simulink model "FFM_Punch"  (R2017a)
settings: Solver=ode3  StartTime=0.0  StopTime=timesteps  FixedStep=data.SIM.Ts  RelTol=1e-3  EnableMultiTasking=on
values from neighbouring files (symbols this model uses):
  data =     [dakota_config.mat]
  downshift_map = data.TCU.upshift.veh_spd_default    [Simulation_results.m]
  upshift_map = data.TCU.upshift.veh_spd_default    [Simulation_results.m]
undefined symbols (not defined in the file or in its folder): air_density, Cd, DiscIntNeverNeededParam, fr_crankshaft, fr_speed_values, g, i_FD, ICE, Low_Ratio, M_Eng_Max, M_Eng_Max_Max, M_Eng_Max_Rpm, mt2m_f, mu_Roll_C0, mu_Roll_C1, mu_Roll_C2, Mv, n_Idle_Eng, Overdrive_Ratio, Re, S_eff_drag, Ts
(part 15 of 15)

== system FFM_Punch/Driver Interface/Driver Model/Driver Pedals Determination/Throttle_Pedal_Determination/RateLimiter ==
  UL : Inport  Tag=Controls_Lib_V1.0  OutDataTypeStr=single  Interpolate=off
  Inp : Inport  Tag=Controls_Lib_V1.0  Port=2  OutDataTypeStr=single  Interpolate=off
  LL : Inport  Tag=Controls_Lib_V1.0  Port=3  OutDataTypeStr=single  Interpolate=off
  AddSub : Sum  Tag=Controls_Lib_V1.0  Inputs=+-  CollapseDim=CollapseDim  AccumDataTypeStr=single  OutMin=OutMin  OutMax=OutMax  OutDataTypeStr=single  RndMeth=Nearest  SampleTime=SampleTime  InputSameDT=on  mask(AddSub){IconShape=rectangular, Inputs=+-, CollapseMode=All dimensions, CollapseDim=1, SampleTime=-1, InputSameDT=on, AccumDataTypeStr=single, OutMin=[], OutMax=[], OutDataTypeStr=single, LockScale=off, RndMeth=Nearest, SaturateOnIntegerOverflow=off}
      mask prompts: IconShape "Icon shape:"; Inputs "List of signs:"; CollapseMode "Sum over:"; CollapseDim "Dimension:"; SampleTime "Sample time (-1 for inherited):"; InputSameDT "Require all inputs to have the same data type"; AccumDataTypeStr "Accumulator data type:"; OutMin "Output minimum:"; OutMax "Output maximum:"; OutDataTypeStr "Output data type:"; LockScale "Lock data type settings against changes by the fixed-point tools"; RndMeth "Integer rounding mode:"; SaturateOnIntegerOverflow "Saturate on integer overflow"
      mask help:
      | Add or subtract inputs.  Specify one of the following:
      | a) string containing + or - for each input port, | for spacer between ports (e.g. ++|-|++)
      | b) scalar, >= 1, specifies the number of input ports to be summed.
      | When there is only one input port, add or subtract elements over all dimensions or one specified dimension
      mask Help: web([fileparts(which('Lib_built')) filesep 'hlp' filesep 'lib_AddSub' '.html'], '-helpbrowser')
      mask TypeOptions IconShape: IconShape
      mask TypeOptions Inputs: Inputs
      mask TypeOptions CollapseMode: CollapseMode
      mask TypeOptions CollapseDim: CollapseDim
      mask TypeOptions SampleTime: SampleTime
      mask TypeOptions InputSameDT: InputSameDT
      mask TypeOptions AccumDataTypeStr: AccumDataTypeStr
      mask TypeOptions OutMin: OutMin
      mask TypeOptions OutMax: OutMax
      mask TypeOptions OutDataTypeStr: OutDataTypeStr
      mask TypeOptions LockScale: LockScale
      mask TypeOptions RndMeth: RndMeth
      mask TypeOptions SaturateOnIntegerOverflow: SaturateOnIntegerOverflow
  AddSub1 : Sum  Tag=Controls_Lib_V1.0  CollapseDim=CollapseDim  AccumDataTypeStr=single  OutMin=OutMin  OutMax=OutMax  OutDataTypeStr=single  RndMeth=Nearest  SampleTime=SampleTime  InputSameDT=on  mask(AddSub){IconShape=rectangular, Inputs=++, CollapseMode=All dimensions, CollapseDim=1, SampleTime=-1, InputSameDT=on, AccumDataTypeStr=single, OutMin=[], OutMax=[], OutDataTypeStr=single, LockScale=off, RndMeth=Nearest, SaturateOnIntegerOverflow=off}
      mask prompts: IconShape "Icon shape:"; Inputs "List of signs:"; CollapseMode "Sum over:"; CollapseDim "Dimension:"; SampleTime "Sample time (-1 for inherited):"; InputSameDT "Require all inputs to have the same data type"; AccumDataTypeStr "Accumulator data type:"; OutMin "Output minimum:"; OutMax "Output maximum:"; OutDataTypeStr "Output data type:"; LockScale "Lock data type settings against changes by the fixed-point tools"; RndMeth "Integer rounding mode:"; SaturateOnIntegerOverflow "Saturate on integer overflow"
      mask help:
      | Add or subtract inputs.  Specify one of the following:
      | a) string containing + or - for each input port, | for spacer between ports (e.g. ++|-|++)
      | b) scalar, >= 1, specifies the number of input ports to be summed.
      | When there is only one input port, add or subtract elements over all dimensions or one specified dimension
      mask Help: web([fileparts(which('Lib_built')) filesep 'hlp' filesep 'lib_AddSub' '.html'], '-helpbrowser')
      mask TypeOptions IconShape: IconShape
      mask TypeOptions Inputs: Inputs
      mask TypeOptions CollapseMode: CollapseMode
      mask TypeOptions CollapseDim: CollapseDim
      mask TypeOptions SampleTime: SampleTime
      mask TypeOptions InputSameDT: InputSameDT
      mask TypeOptions AccumDataTypeStr: AccumDataTypeStr
      mask TypeOptions OutMin: OutMin
      mask TypeOptions OutMax: OutMax
      mask TypeOptions OutDataTypeStr: OutDataTypeStr
      mask TypeOptions LockScale: LockScale
      mask TypeOptions RndMeth: RndMeth
      mask TypeOptions SaturateOnIntegerOverflow: SaturateOnIntegerOverflow
  AddSub2 : Sum  Tag=Controls_Lib_V1.0  CollapseDim=CollapseDim  AccumDataTypeStr=single  OutMin=OutMin  OutMax=OutMax  OutDataTypeStr=single  RndMeth=Nearest  SampleTime=SampleTime  InputSameDT=on  mask(AddSub){IconShape=rectangular, Inputs=++, CollapseMode=All dimensions, CollapseDim=1, SampleTime=-1, InputSameDT=on, AccumDataTypeStr=single, OutMin=[], OutMax=[], OutDataTypeStr=single, LockScale=off, RndMeth=Nearest, SaturateOnIntegerOverflow=off}
      mask prompts: IconShape "Icon shape:"; Inputs "List of signs:"; CollapseMode "Sum over:"; CollapseDim "Dimension:"; SampleTime "Sample time (-1 for inherited):"; InputSameDT "Require all inputs to have the same data type"; AccumDataTypeStr "Accumulator data type:"; OutMin "Output minimum:"; OutMax "Output maximum:"; OutDataTypeStr "Output data type:"; LockScale "Lock data type settings against changes by the fixed-point tools"; RndMeth "Integer rounding mode:"; SaturateOnIntegerOverflow "Saturate on integer overflow"
      mask help:
      | Add or subtract inputs.  Specify one of the following:
      | a) string containing + or - for each input port, | for spacer between ports (e.g. ++|-|++)
      | b) scalar, >= 1, specifies the number of input ports to be summed.
      | When there is only one input port, add or subtract elements over all dimensions or one specified dimension
      mask Help: web([fileparts(which('Lib_built')) filesep 'hlp' filesep 'lib_AddSub' '.html'], '-helpbrowser')
      mask TypeOptions IconShape: IconShape
      mask TypeOptions Inputs: Inputs
      mask TypeOptions CollapseMode: CollapseMode
      mask TypeOptions CollapseDim: CollapseDim
      mask TypeOptions SampleTime: SampleTime
      mask TypeOptions InputSameDT: InputSameDT
      mask TypeOptions AccumDataTypeStr: AccumDataTypeStr
      mask TypeOptions OutMin: OutMin
      mask TypeOptions OutMax: OutMax
      mask TypeOptions OutDataTypeStr: OutDataTypeStr
      mask TypeOptions LockScale: LockScale
      mask TypeOptions RndMeth: RndMeth
      mask TypeOptions SaturateOnIntegerOverflow: SaturateOnIntegerOverflow
  AddSub3 : Sum  Tag=Controls_Lib_V1.0  Inputs=-+  CollapseDim=CollapseDim  AccumDataTypeStr=single  OutMin=OutMin  OutMax=OutMax  OutDataTypeStr=single  RndMeth=Nearest  SampleTime=SampleTime  InputSameDT=on  mask(AddSub){IconShape=rectangular, Inputs=-+, CollapseMode=All dimensions, CollapseDim=1, SampleTime=-1, InputSameDT=on, AccumDataTypeStr=single, OutMin=[], OutMax=[], OutDataTypeStr=single, LockScale=off, RndMeth=Nearest, SaturateOnIntegerOverflow=off}
      mask prompts: IconShape "Icon shape:"; Inputs "List of signs:"; CollapseMode "Sum over:"; CollapseDim "Dimension:"; SampleTime "Sample time (-1 for inherited):"; InputSameDT "Require all inputs to have the same data type"; AccumDataTypeStr "Accumulator data type:"; OutMin "Output minimum:"; OutMax "Output maximum:"; OutDataTypeStr "Output data type:"; LockScale "Lock data type settings against changes by the fixed-point tools"; RndMeth "Integer rounding mode:"; SaturateOnIntegerOverflow "Saturate on integer overflow"
      mask help:
      | Add or subtract inputs.  Specify one of the following:
      | a) string containing + or - for each input port, | for spacer between ports (e.g. ++|-|++)
      | b) scalar, >= 1, specifies the number of input ports to be summed.
      | When there is only one input port, add or subtract elements over all dimensions or one specified dimension
      mask Help: web([fileparts(which('Lib_built')) filesep 'hlp' filesep 'lib_AddSub' '.html'], '-helpbrowser')
      mask TypeOptions IconShape: IconShape
      mask TypeOptions Inputs: Inputs
      mask TypeOptions CollapseMode: CollapseMode
      mask TypeOptions CollapseDim: CollapseDim
      mask TypeOptions SampleTime: SampleTime
      mask TypeOptions InputSameDT: InputSameDT
      mask TypeOptions AccumDataTypeStr: AccumDataTypeStr
      mask TypeOptions OutMin: OutMin
      mask TypeOptions OutMax: OutMax
      mask TypeOptions OutDataTypeStr: OutDataTypeStr
      mask TypeOptions LockScale: LockScale
      mask TypeOptions RndMeth: RndMeth
      mask TypeOptions SaturateOnIntegerOverflow: SaturateOnIntegerOverflow
  Constant : Constant  Tag=Controls_Lib_V1.0  Value=Value  VectorParams1D=off  OutMin=OutMin  OutMax=OutMax  OutDataTypeStr=Inherit: Inherit via back propagation  SampleTime=SampleTime  FramePeriod=FramePeriod  mask(Constant){Value=0.5, VectorParams1D=off, SampleTime=-1, FramePeriod=inf, OutMin=[], OutMax=[], OutDataTypeStr=Inherit: Inherit via back propagation, LockScale=off}
      mask prompts: Value "Constant value:"; VectorParams1D "Interpret vector parameters as 1-D"; SampleTime "Sample time:"; FramePeriod "Frame period:"; OutMin "Output minimum:"; OutMax "Output maximum:"; OutDataTypeStr "Output data type:"; LockScale "Lock output data type setting against changes by the fixed-point tools"
      mask help: Output the constant specified by the 'Constant value' parameter.
      mask TypeOptions Value: Value
      mask TypeOptions VectorParams1D: VectorParams1D
      mask TypeOptions SampleTime: SampleTime
      mask TypeOptions FramePeriod: FramePeriod
      mask TypeOptions OutMin: OutMin
      mask TypeOptions OutMax: OutMax
      mask TypeOptions OutDataTypeStr: OutDataTypeStr
      mask TypeOptions LockScale: LockScale
      mask Display: disp(get_param(gcb,'Value'))
  Constant1 : Constant  Tag=Controls_Lib  Description=constant  Value=Value  OutMin=OutMin  OutMax=OutMax  OutDataTypeStr=single  SampleTime=SampleTime  FramePeriod=FramePeriod  mask(Constant){Value=1, VectorParams1D=on, SampleTime=-1, FramePeriod=inf, OutMin=[], OutMax=[], OutDataTypeStr=single, LockScale=off}
      mask prompts: Value "Constant value:"; VectorParams1D "Interpret vector parameters as 1-D"; SampleTime "Sample time:"; FramePeriod "Frame period:"; OutMin "Output minimum:"; OutMax "Output maximum:"; OutDataTypeStr "Output data type:"; LockScale "Lock output data type setting against changes by the fixed-point tools"
      mask help: Output the constant specified by the 'Constant value' parameter.
      mask TypeOptions Value: Value
      mask TypeOptions VectorParams1D: VectorParams1D
      mask TypeOptions SampleTime: SampleTime
      mask TypeOptions FramePeriod: FramePeriod
      mask TypeOptions OutMin: OutMin
      mask TypeOptions OutMax: OutMax
      mask TypeOptions OutDataTypeStr: OutDataTypeStr
      mask TypeOptions LockScale: LockScale
      mask Display: disp(get_param(gcb,'Value'))
  Delay : Delay  Tag=Controls_Lib_V1.0  DelayLength=DelayLength  DelayLengthUpperLimit=DelayLengthUpperLimit  InitialConditionSource=Input port  InitialCondition=InitialCondition  SampleTime=SampleTime  mask(Delay){DelayLengthSource=Dialog, DelayLength=1, DelayLengthUpperLimit=100, InitialConditionSource=Input port, InitialCondition=0.0, ExternalReset=None, PreventDirectFeedthrough=off, DiagnosticForOutOfRangeDelayLength=None, RemoveProtectionDelayLength=off, InputProcessing=Elements as channels (sample based), UseCircularBuffer=off, SampleTime=-1, StateName=, StateMustResolveToSignalObject=off, CodeGenStateStorageClass=Auto, CodeGenStateStorageTypeQualifier=}
      mask prompts: DelayLengthSource "Delay length source:"; DelayLength "Delay length:"; DelayLengthUpperLimit "Delay upper limit:"; InitialConditionSource "Initial condition source:"; InitialCondition "Initial condition:"; ExternalReset "External reset:"; PreventDirectFeedthrough "Prevent direct feedthrough by increasing delay length to lower limit"; DiagnosticForOutOfRangeDelayLength "Diagnostic for out-of-range delay length:"; RemoveProtectionDelayLength "Remove protection against out-of-range delay length in generated code"; InputProcessing "Input processing:"; UseCircularBuffer "Use circular buffer for state"; SampleTime "Sample time (-1 for inherited):"; StateName "State name:"; StateMustResolveToSignalObject "State name must resolve to Simulink signal object"; CodeGenStateStorageClass "Code generation storage class:"; CodeGenStateStorageTypeQualifier "Code generation storage type qualifier:"
      mask help: Delay input by a fixed or variable number of samples. The initial output of the delay block is specified by the external input x0.
      settings: InputPortMap=u0,p4
      mask TypeOptions DelayLengthSource: DelayLengthSource
      mask TypeOptions DelayLength: DelayLength
      mask TypeOptions DelayLengthUpperLimit: DelayLengthUpperLimit
      mask TypeOptions InitialConditionSource: InitialConditionSource
      mask TypeOptions InitialCondition: InitialCondition
      mask TypeOptions ExternalReset: ExternalReset
      mask TypeOptions PreventDirectFeedthrough: PreventDirectFeedthrough
      mask TypeOptions DiagnosticForOutOfRangeDelayLength: DiagnosticForOutOfRangeDelayLength
      mask TypeOptions RemoveProtectionDelayLength: RemoveProtectionDelayLength
      mask TypeOptions InputProcessing: InputProcessing
      mask TypeOptions UseCircularBuffer: UseCircularBuffer
      mask TypeOptions SampleTime: SampleTime
      mask TypeOptions StateName: StateName
      mask TypeOptions StateMustResolveToSignalObject: StateMustResolveToSignalObject
      mask TypeOptions CodeGenStateStorageClass: CodeGenStateStorageClass
      mask TypeOptions CodeGenStateStorageTypeQualifier: CodeGenStateStorageTypeQualifier
  MulDiv : Product  Tag=Controls_Lib_V1.0  Inputs=*/  CollapseDim=CollapseDim  OutMin=OutMin  OutMax=OutMax  OutDataTypeStr=single  SampleTime=SampleTime  InputSameDT=on  mask(MulDiv){Inputs=*/, Multiplication=Element-wise(.*), CollapseMode=All dimensions, CollapseDim=1, SampleTime=-1, InputSameDT=on, OutMin=[], OutMax=[], OutDataTypeStr=single, LockScale=off, RndMeth=Floor, SaturateOnIntegerOverflow=off}
      mask prompts: Inputs "Number of inputs:"; CollapseMode "Multiply over:"; CollapseDim "Dimension:"; SampleTime "Sample time (-1 for inherited):"; InputSameDT "Require all inputs to have the same data type"; OutMin "Output minimum:"; OutMax "Output maximum:"; OutDataTypeStr "Output data type:"; LockScale "Lock output data type setting against changes by the fixed-point tools"; RndMeth "Integer rounding mode:"; SaturateOnIntegerOverflow "Saturate on integer overflow"
      mask help:
      | Multiply or divide inputs element-wise. Specify one of the following:
      |  a) * or / for each input port. For example, **/* performs the operation 'u1*u2/u3*u4'.
      |  b) scalar specifies the number of input ports to be multiplied.
      | If there is only one input port and the Multiplication parameter is set to Element-wise(.*), a single * or / collapses the input signal using the specified operation.
      mask Help: web([fileparts(which('Lib_built')) filesep 'hlp' filesep 'lib_MulDiv' '.html'], '-helpbrowser')
      mask TypeOptions Inputs: Inputs
      mask TypeOptions Multiplication: Multiplication
      mask TypeOptions CollapseMode: CollapseMode
      mask TypeOptions CollapseDim: CollapseDim
      mask TypeOptions SampleTime: SampleTime
      mask TypeOptions InputSameDT: InputSameDT
      mask TypeOptions OutMin: OutMin
      mask TypeOptions OutMax: OutMax
      mask TypeOptions OutDataTypeStr: OutDataTypeStr
      mask TypeOptions LockScale: LockScale
      mask TypeOptions RndMeth: RndMeth
      mask TypeOptions SaturateOnIntegerOverflow: SaturateOnIntegerOverflow
  MulDiv1 : Product  Tag=Controls_Lib_V1.0  Inputs=**  CollapseDim=CollapseDim  OutMin=OutMin  OutMax=OutMax  OutDataTypeStr=single  SampleTime=SampleTime  InputSameDT=on  mask(MulDiv){Inputs=**, Multiplication=Element-wise(.*), CollapseMode=All dimensions, CollapseDim=1, SampleTime=-1, InputSameDT=on, OutMin=[], OutMax=[], OutDataTypeStr=single, LockScale=off, RndMeth=Floor, SaturateOnIntegerOverflow=off}
      mask prompts: Inputs "Number of inputs:"; CollapseMode "Multiply over:"; CollapseDim "Dimension:"; SampleTime "Sample time (-1 for inherited):"; InputSameDT "Require all inputs to have the same data type"; OutMin "Output minimum:"; OutMax "Output maximum:"; OutDataTypeStr "Output data type:"; LockScale "Lock output data type setting against changes by the fixed-point tools"; RndMeth "Integer rounding mode:"; SaturateOnIntegerOverflow "Saturate on integer overflow"
      mask help:
      | Multiply or divide inputs element-wise. Specify one of the following:
      |  a) * or / for each input port. For example, **/* performs the operation 'u1*u2/u3*u4'.
      |  b) scalar specifies the number of input ports to be multiplied.
      | If there is only one input port and the Multiplication parameter is set to Element-wise(.*), a single * or / collapses the input signal using the specified operation.
      mask Help: web([fileparts(which('Lib_built')) filesep 'hlp' filesep 'lib_MulDiv' '.html'], '-helpbrowser')
      mask TypeOptions Inputs: Inputs
      mask TypeOptions Multiplication: Multiplication
      mask TypeOptions CollapseMode: CollapseMode
      mask TypeOptions CollapseDim: CollapseDim
      mask TypeOptions SampleTime: SampleTime
      mask TypeOptions InputSameDT: InputSameDT
      mask TypeOptions OutMin: OutMin
      mask TypeOptions OutMax: OutMax
      mask TypeOptions OutDataTypeStr: OutDataTypeStr
      mask TypeOptions LockScale: LockScale
      mask TypeOptions RndMeth: RndMeth
      mask TypeOptions SaturateOnIntegerOverflow: SaturateOnIntegerOverflow
  MulDiv2 : Product  Tag=Controls_Lib_V1.0  Inputs=***  CollapseDim=CollapseDim  OutMin=OutMin  OutMax=OutMax  OutDataTypeStr=single  SampleTime=SampleTime  InputSameDT=on  mask(MulDiv){Inputs=***, Multiplication=Element-wise(.*), CollapseMode=All dimensions, CollapseDim=1, SampleTime=-1, InputSameDT=on, OutMin=[], OutMax=[], OutDataTypeStr=single, LockScale=off, RndMeth=Floor, SaturateOnIntegerOverflow=off}
      mask prompts: Inputs "Number of inputs:"; CollapseMode "Multiply over:"; CollapseDim "Dimension:"; SampleTime "Sample time (-1 for inherited):"; InputSameDT "Require all inputs to have the same data type"; OutMin "Output minimum:"; OutMax "Output maximum:"; OutDataTypeStr "Output data type:"; LockScale "Lock output data type setting against changes by the fixed-point tools"; RndMeth "Integer rounding mode:"; SaturateOnIntegerOverflow "Saturate on integer overflow"
      mask help:
      | Multiply or divide inputs element-wise. Specify one of the following:
      |  a) * or / for each input port. For example, **/* performs the operation 'u1*u2/u3*u4'.
      |  b) scalar specifies the number of input ports to be multiplied.
      | If there is only one input port and the Multiplication parameter is set to Element-wise(.*), a single * or / collapses the input signal using the specified operation.
      mask Help: web([fileparts(which('Lib_built')) filesep 'hlp' filesep 'lib_MulDiv' '.html'], '-helpbrowser')
      mask TypeOptions Inputs: Inputs
      mask TypeOptions Multiplication: Multiplication
      mask TypeOptions CollapseMode: CollapseMode
      mask TypeOptions CollapseDim: CollapseDim
      mask TypeOptions SampleTime: SampleTime
      mask TypeOptions InputSameDT: InputSameDT
      mask TypeOptions OutMin: OutMin
      mask TypeOptions OutMax: OutMax
      mask TypeOptions OutDataTypeStr: OutDataTypeStr
      mask TypeOptions LockScale: LockScale
      mask TypeOptions RndMeth: RndMeth
      mask TypeOptions SaturateOnIntegerOverflow: SaturateOnIntegerOverflow
  MulDiv3 : Product  Tag=Controls_Lib_V1.0  Inputs=*/  CollapseDim=CollapseDim  OutMin=OutMin  OutMax=OutMax  OutDataTypeStr=single  SampleTime=SampleTime  InputSameDT=on  mask(MulDiv){Inputs=*/, Multiplication=Element-wise(.*), CollapseMode=All dimensions, CollapseDim=1, SampleTime=-1, InputSameDT=on, OutMin=[], OutMax=[], OutDataTypeStr=single, LockScale=off, RndMeth=Floor, SaturateOnIntegerOverflow=off}
      mask prompts: Inputs "Number of inputs:"; CollapseMode "Multiply over:"; CollapseDim "Dimension:"; SampleTime "Sample time (-1 for inherited):"; InputSameDT "Require all inputs to have the same data type"; OutMin "Output minimum:"; OutMax "Output maximum:"; OutDataTypeStr "Output data type:"; LockScale "Lock output data type setting against changes by the fixed-point tools"; RndMeth "Integer rounding mode:"; SaturateOnIntegerOverflow "Saturate on integer overflow"
      mask help:
      | Multiply or divide inputs element-wise. Specify one of the following:
      |  a) * or / for each input port. For example, **/* performs the operation 'u1*u2/u3*u4'.
      |  b) scalar specifies the number of input ports to be multiplied.
      | If there is only one input port and the Multiplication parameter is set to Element-wise(.*), a single * or / collapses the input signal using the specified operation.
      mask Help: web([fileparts(which('Lib_built')) filesep 'hlp' filesep 'lib_MulDiv' '.html'], '-helpbrowser')
      mask TypeOptions Inputs: Inputs
      mask TypeOptions Multiplication: Multiplication
      mask TypeOptions CollapseMode: CollapseMode
      mask TypeOptions CollapseDim: CollapseDim
      mask TypeOptions SampleTime: SampleTime
      mask TypeOptions InputSameDT: InputSameDT
      mask TypeOptions OutMin: OutMin
      mask TypeOptions OutMax: OutMax
      mask TypeOptions OutDataTypeStr: OutDataTypeStr
      mask TypeOptions LockScale: LockScale
      mask TypeOptions RndMeth: RndMeth
      mask TypeOptions SaturateOnIntegerOverflow: SaturateOnIntegerOverflow
  SatChck : Subsystem  mask(SATURATION){}
      mask help:
      | The Saturation with Check block imposes upper and lower limits on an input signal. If the input signal is outside of these limits, saturation flag shall be raised.
      |
      | The upper limit (Max) shall be  greater than the lower limit (Min) for the saturation block to work as intended.
      mask Help: web([fileparts(which('Lib_discontious')) filesep 'hlp' filesep 'lib_SatChck.html'], '-helpbrowser')
      mask Display: plot([0 1 2 3 4 5],[0 0 0 1 1 1],[0 5],[0.5 0.5],[2.5 2.5],[0 1])
  TsInverse : SampleTimeMath  TsampMathOp=1/Ts Only  weightValue=weightValue  OutDataTypeStr=Inherit: Inherit via back propagation  mask(Sample time block){TsampMathOp=1/Ts Only, weightValue=1, TsampMathImp=Online Calculations, OutDataTypeStr=Inherit: Inherit via back propagation, RndMeth=Floor, SaturateOnIntegerOverflow=off}
      mask prompts: TsampMathOp "Operation:"; weightValue "Weight value:"; TsampMathImp "Implement using:"; OutDataTypeStr "Output data type:"; RndMeth "Integer rounding mode:"; SaturateOnIntegerOverflow "Saturate on integer overflow"
      mask help: 1 divided by the Sample time of the input signal
      mask Help: web([fileparts(which('Lib_built')) filesep 'hlp' filesep 'lib_TsInv' '.html'], '-helpbrowser')
      mask TypeOptions TsampMathOp: TsampMathOp
      mask TypeOptions weightValue: weightValue
      mask TypeOptions TsampMathImp: TsampMathImp
      mask TypeOptions OutDataTypeStr: OutDataTypeStr
      mask TypeOptions RndMeth: RndMeth
      mask TypeOptions SaturateOnIntegerOverflow: SaturateOnIntegerOverflow
  Out : Outport  Tag=Controls_Lib_V1.0  OutDataTypeStr=single  InitialOutput=0
  Issat : Outport  Tag=Controls_Lib_V1.0  Port=2  OutDataTypeStr=boolean  InitialOutput=0
  wires:
  MulDiv3/1 -> [Ts]
  TsInverse/1 -> MulDiv3/2
  Constant1/1 -> MulDiv3/1
  [Init] -> Delay/2
  Delay/1 -> [OutPrev]
  AddSub3/1 -> [Init]
  MulDiv2/1 -> AddSub3/1
  [Inp] -> AddSub3/2
  Constant/1 -> MulDiv2/3
  AddSub2/1 -> MulDiv2/2
  [LL] -> AddSub2/2
  [UL] -> AddSub2/1
  AddSub1/1 -> Delay/1, Out/1
  [Ts] -> MulDiv1/1
  [OutPrev] -> AddSub1/2
  MulDiv1/1 -> AddSub1/1
  SatChck/1(ValSat) -> MulDiv1/2
  MulDiv/1 -> SatChck/2(Inp)
  [Ts] -> MulDiv2/1, MulDiv/2
  AddSub/1 -> MulDiv/1
  SatChck/2(IsSat) -> Issat/1
  [LL] -> SatChck/3(Min)
  [UL] -> SatChck/1(Max)
  [OutPrev] -> AddSub/2
  [Inp] -> AddSub/1
  LL/1 -> [LL]
  Inp/1 -> TsInverse/1, [Inp]
  UL/1 -> [UL]

== system FFM_Punch/Driver Interface/Driver Model/Final Pedal Coordination/RateLimiter/SatChck ==
  Max : Inport  Tag=Controls_Lib_V1.0  OutDataTypeStr=single  Interpolate=off
  Inp : Inport  Tag=Controls_Lib_V1.0  Port=2  OutDataTypeStr=single  Interpolate=off
  Min : Inport  Tag=Controls_Lib_V1.0  Port=3  OutDataTypeStr=single  Interpolate=off
  MinMax : MinMax  Tag=Controls_Lib_V1.0  Inputs=Inputs  OutMin=OutMin  OutMax=OutMax  OutDataTypeStr=single  RndMeth=Zero  SampleTime=SampleTime  InputSameDT=on  mask(MinMax){Function=min, Inputs=2, ZeroCross=on, SampleTime=-1, InputSameDT=on, OutMin=[], OutMax=[], OutDataTypeStr=single, LockScale=off, RndMeth=Zero, SaturateOnIntegerOverflow=off}
      mask prompts: Inputs "Number of input ports:"; ZeroCross "Enable zero-crossing detection"; SampleTime "Sample time (-1 for inherited):"; InputSameDT "Require all inputs to have the same data type"; OutMin "Output minimum:"; OutMax "Output maximum:"; OutDataTypeStr "Output data type:"; LockScale "Lock output data type setting against changes by the fixed-point tools"; RndMeth "Integer rounding mode:"; SaturateOnIntegerOverflow "Saturate on integer overflow"
      mask help: Output min or max of input. For a single input, operators are applied across the input vector. For multiple inputs, operators are applied across the inputs.
      mask Help: web([fileparts(which('Lib_built')) filesep 'hlp' filesep 'lib_MinMax' '.html'], '-helpbrowser')
      mask TypeOptions Function: Function
      mask TypeOptions Inputs: Inputs
      mask TypeOptions ZeroCross: ZeroCross
      mask TypeOptions SampleTime: SampleTime
      mask TypeOptions InputSameDT: InputSameDT
      mask TypeOptions OutMin: OutMin
      mask TypeOptions OutMax: OutMax
      mask TypeOptions OutDataTypeStr: OutDataTypeStr
      mask TypeOptions LockScale: LockScale
      mask TypeOptions RndMeth: RndMeth
      mask TypeOptions SaturateOnIntegerOverflow: SaturateOnIntegerOverflow
  MinMax1 : MinMax  Tag=Controls_Lib_V1.0  Function=max  Inputs=Inputs  OutMin=OutMin  OutMax=OutMax  OutDataTypeStr=single  RndMeth=Zero  SampleTime=SampleTime  InputSameDT=on  mask(MinMax){Function=max, Inputs=2, ZeroCross=on, SampleTime=-1, InputSameDT=on, OutMin=[], OutMax=[], OutDataTypeStr=single, LockScale=off, RndMeth=Zero, SaturateOnIntegerOverflow=off}
      mask prompts: Inputs "Number of input ports:"; ZeroCross "Enable zero-crossing detection"; SampleTime "Sample time (-1 for inherited):"; InputSameDT "Require all inputs to have the same data type"; OutMin "Output minimum:"; OutMax "Output maximum:"; OutDataTypeStr "Output data type:"; LockScale "Lock output data type setting against changes by the fixed-point tools"; RndMeth "Integer rounding mode:"; SaturateOnIntegerOverflow "Saturate on integer overflow"
      mask help: Output min or max of input. For a single input, operators are applied across the input vector. For multiple inputs, operators are applied across the inputs.
      mask Help: web([fileparts(which('Lib_built')) filesep 'hlp' filesep 'lib_MinMax' '.html'], '-helpbrowser')
      mask TypeOptions Function: Function
      mask TypeOptions Inputs: Inputs
      mask TypeOptions ZeroCross: ZeroCross
      mask TypeOptions SampleTime: SampleTime
      mask TypeOptions InputSameDT: InputSameDT
      mask TypeOptions OutMin: OutMin
      mask TypeOptions OutMax: OutMax
      mask TypeOptions OutDataTypeStr: OutDataTypeStr
      mask TypeOptions LockScale: LockScale
      mask TypeOptions RndMeth: RndMeth
      mask TypeOptions SaturateOnIntegerOverflow: SaturateOnIntegerOverflow
  RelationalOperator : RelationalOperator  Tag=Controls_Lib_V1.0  Operator=~=  OutDataTypeStr=boolean  SampleTime=SampleTime  RndMeth=Nearest  InputSameDT=on  mask(Relational operator){Operator=~=, ZeroCross=on, SampleTime=-1, InputSameDT=on, OutDataTypeStr=boolean}
      mask prompts: Operator "Relational operator:"; ZeroCross "Enable zero-crossing detection"; SampleTime "Sample time (-1 for inherited):"; InputSameDT "Require all inputs to have the same data type"; OutDataTypeStr "Output data type:"
      mask help: Applies the selected relational operator to the inputs and outputs the result. The top (or left) input corresponds to the first operand.
      mask Help: web([fileparts(which('Lib_built')) filesep 'hlp' filesep 'lib_Relational' '.html'], '-helpbrowser')
      mask TypeOptions Operator: Operator
      mask TypeOptions ZeroCross: ZeroCross
      mask TypeOptions SampleTime: SampleTime
      mask TypeOptions InputSameDT: InputSameDT
      mask TypeOptions OutDataTypeStr: OutDataTypeStr
  ValSat : Outport  Tag=Controls_Lib_V1.0  OutDataTypeStr=single  InitialOutput=0
  IsSat : Outport  Tag=Controls_Lib_V1.0  Port=2  OutDataTypeStr=boolean  InitialOutput=0
  wires:
  Max/1 -> MinMax/1
  Inp/1 -> MinMax/2, RelationalOperator/2
  MinMax/1 -> MinMax1/1
  Min/1 -> MinMax1/2
  MinMax1/1 -> RelationalOperator/1, ValSat/1
  RelationalOperator/1 -> IsSat/1

== system FFM_Punch/Controller/F02_03_03_05_Raw_Gear_Target_Auto_Mode/F02_03_03_05_09_Final_Raw_Gear_Target_Auto_Mode/TurnOnDelay1/Timer/falling_edge ==
  Signal : Inport
  Logical Operator : Logic  Tag=struct('inputs','2','comment',struct('text','','placement',1),'logdata',struct('maxnumvals',inf,'plotchannels',[],'loggingmode',3,'channels',1),'operator','AND','output',struct('variable','','description','','name','$S_$B','address','','class','default','type','Bool','unit',''),'scalingvalid',0,'date',733067.68453166669)  OutDataTypeStr=boolean
  Logical Operator1 : Logic  Tag=struct('inputs','1','comment',struct('text','','placement',1),'logdata',struct('maxnumvals',inf,'plotchannels',[],'loggingmode',3,'channels',1),'operator','NOT','output',struct('variable','','description','','name','$S_$B','address','','class','default','type','Bool','unit',''),'scalingvalid',0,'date',733067.68453201384)  Operator=NOT  Inputs=1  OutDataTypeStr=boolean
  UnitDelay : UnitDelay  SampleTime=-1
      settings: AttributesFormatString=Te = %<SampleTime>\nIni=%<X0>
  Out : Outport
  wires:
  UnitDelay/1 -> Logical Operator/2
  Logical Operator1/1 -> Logical Operator/1
  Signal/1 -> UnitDelay/1, Logical Operator1/1
  Logical Operator/1 -> Out/1

== system FFM_Punch/Controller/F02_03_03_05_Raw_Gear_Target_Auto_Mode/F02_03_03_05_09_Final_Raw_Gear_Target_Auto_Mode/TurnOnDelay2/Timer/falling_edge ==
  Signal : Inport
  Logical Operator : Logic  Tag=struct('inputs','2','comment',struct('text','','placement',1),'logdata',struct('maxnumvals',inf,'plotchannels',[],'loggingmode',3,'channels',1),'operator','AND','output',struct('variable','','description','','name','$S_$B','address','','class','default','type','Bool','unit',''),'scalingvalid',0,'date',733067.68453166669)  OutDataTypeStr=boolean
  Logical Operator1 : Logic  Tag=struct('inputs','1','comment',struct('text','','placement',1),'logdata',struct('maxnumvals',inf,'plotchannels',[],'loggingmode',3,'channels',1),'operator','NOT','output',struct('variable','','description','','name','$S_$B','address','','class','default','type','Bool','unit',''),'scalingvalid',0,'date',733067.68453201384)  Operator=NOT  Inputs=1  OutDataTypeStr=boolean
  UnitDelay : UnitDelay  SampleTime=-1
      settings: AttributesFormatString=Te = %<SampleTime>\nIni=%<X0>
  Out : Outport
  wires:
  UnitDelay/1 -> Logical Operator/2
  Logical Operator1/1 -> Logical Operator/1
  Signal/1 -> UnitDelay/1, Logical Operator1/1
  Logical Operator/1 -> Out/1

== system FFM_Punch/Driver Interface/Driver Model/Driver Pedals Determination/Preliminary_Calculations/RateLimiter/SatChck ==
  Max : Inport  Tag=Controls_Lib_V1.0  OutDataTypeStr=single  Interpolate=off
  Inp : Inport  Tag=Controls_Lib_V1.0  Port=2  OutDataTypeStr=single  Interpolate=off
  Min : Inport  Tag=Controls_Lib_V1.0  Port=3  OutDataTypeStr=single  Interpolate=off
  MinMax : MinMax  Tag=Controls_Lib_V1.0  Inputs=Inputs  OutMin=OutMin  OutMax=OutMax  OutDataTypeStr=single  RndMeth=Zero  SampleTime=SampleTime  InputSameDT=on  mask(MinMax){Function=min, Inputs=2, ZeroCross=on, SampleTime=-1, InputSameDT=on, OutMin=[], OutMax=[], OutDataTypeStr=single, LockScale=off, RndMeth=Zero, SaturateOnIntegerOverflow=off}
      mask prompts: Inputs "Number of input ports:"; ZeroCross "Enable zero-crossing detection"; SampleTime "Sample time (-1 for inherited):"; InputSameDT "Require all inputs to have the same data type"; OutMin "Output minimum:"; OutMax "Output maximum:"; OutDataTypeStr "Output data type:"; LockScale "Lock output data type setting against changes by the fixed-point tools"; RndMeth "Integer rounding mode:"; SaturateOnIntegerOverflow "Saturate on integer overflow"
      mask help: Output min or max of input. For a single input, operators are applied across the input vector. For multiple inputs, operators are applied across the inputs.
      mask Help: web([fileparts(which('Lib_built')) filesep 'hlp' filesep 'lib_MinMax' '.html'], '-helpbrowser')
      mask TypeOptions Function: Function
      mask TypeOptions Inputs: Inputs
      mask TypeOptions ZeroCross: ZeroCross
      mask TypeOptions SampleTime: SampleTime
      mask TypeOptions InputSameDT: InputSameDT
      mask TypeOptions OutMin: OutMin
      mask TypeOptions OutMax: OutMax
      mask TypeOptions OutDataTypeStr: OutDataTypeStr
      mask TypeOptions LockScale: LockScale
      mask TypeOptions RndMeth: RndMeth
      mask TypeOptions SaturateOnIntegerOverflow: SaturateOnIntegerOverflow
  MinMax1 : MinMax  Tag=Controls_Lib_V1.0  Function=max  Inputs=Inputs  OutMin=OutMin  OutMax=OutMax  OutDataTypeStr=single  RndMeth=Zero  SampleTime=SampleTime  InputSameDT=on  mask(MinMax){Function=max, Inputs=2, ZeroCross=on, SampleTime=-1, InputSameDT=on, OutMin=[], OutMax=[], OutDataTypeStr=single, LockScale=off, RndMeth=Zero, SaturateOnIntegerOverflow=off}
      mask prompts: Inputs "Number of input ports:"; ZeroCross "Enable zero-crossing detection"; SampleTime "Sample time (-1 for inherited):"; InputSameDT "Require all inputs to have the same data type"; OutMin "Output minimum:"; OutMax "Output maximum:"; OutDataTypeStr "Output data type:"; LockScale "Lock output data type setting against changes by the fixed-point tools"; RndMeth "Integer rounding mode:"; SaturateOnIntegerOverflow "Saturate on integer overflow"
      mask help: Output min or max of input. For a single input, operators are applied across the input vector. For multiple inputs, operators are applied across the inputs.
      mask Help: web([fileparts(which('Lib_built')) filesep 'hlp' filesep 'lib_MinMax' '.html'], '-helpbrowser')
      mask TypeOptions Function: Function
      mask TypeOptions Inputs: Inputs
      mask TypeOptions ZeroCross: ZeroCross
      mask TypeOptions SampleTime: SampleTime
      mask TypeOptions InputSameDT: InputSameDT
      mask TypeOptions OutMin: OutMin
      mask TypeOptions OutMax: OutMax
      mask TypeOptions OutDataTypeStr: OutDataTypeStr
      mask TypeOptions LockScale: LockScale
      mask TypeOptions RndMeth: RndMeth
      mask TypeOptions SaturateOnIntegerOverflow: SaturateOnIntegerOverflow
  RelationalOperator : RelationalOperator  Tag=Controls_Lib_V1.0  Operator=~=  OutDataTypeStr=boolean  SampleTime=SampleTime  RndMeth=Nearest  InputSameDT=on  mask(Relational operator){Operator=~=, ZeroCross=on, SampleTime=-1, InputSameDT=on, OutDataTypeStr=boolean}
      mask prompts: Operator "Relational operator:"; ZeroCross "Enable zero-crossing detection"; SampleTime "Sample time (-1 for inherited):"; InputSameDT "Require all inputs to have the same data type"; OutDataTypeStr "Output data type:"
      mask help: Applies the selected relational operator to the inputs and outputs the result. The top (or left) input corresponds to the first operand.
      mask Help: web([fileparts(which('Lib_built')) filesep 'hlp' filesep 'lib_Relational' '.html'], '-helpbrowser')
      mask TypeOptions Operator: Operator
      mask TypeOptions ZeroCross: ZeroCross
      mask TypeOptions SampleTime: SampleTime
      mask TypeOptions InputSameDT: InputSameDT
      mask TypeOptions OutDataTypeStr: OutDataTypeStr
  ValSat : Outport  Tag=Controls_Lib_V1.0  OutDataTypeStr=single  InitialOutput=0
  IsSat : Outport  Tag=Controls_Lib_V1.0  Port=2  OutDataTypeStr=boolean  InitialOutput=0
  wires:
  Max/1 -> MinMax/1
  Inp/1 -> MinMax/2, RelationalOperator/2
  MinMax/1 -> MinMax1/1
  Min/1 -> MinMax1/2
  MinMax1/1 -> RelationalOperator/1, ValSat/1
  RelationalOperator/1 -> IsSat/1

== system FFM_Punch/Driver Interface/Driver Model/Driver Pedals Determination/Throttle_Pedal_Determination/RateLimiter/SatChck ==
  Max : Inport  Tag=Controls_Lib_V1.0  OutDataTypeStr=single  Interpolate=off
  Inp : Inport  Tag=Controls_Lib_V1.0  Port=2  OutDataTypeStr=single  Interpolate=off
  Min : Inport  Tag=Controls_Lib_V1.0  Port=3  OutDataTypeStr=single  Interpolate=off
  MinMax : MinMax  Tag=Controls_Lib_V1.0  Inputs=Inputs  OutMin=OutMin  OutMax=OutMax  OutDataTypeStr=single  RndMeth=Zero  SampleTime=SampleTime  InputSameDT=on  mask(MinMax){Function=min, Inputs=2, ZeroCross=on, SampleTime=-1, InputSameDT=on, OutMin=[], OutMax=[], OutDataTypeStr=single, LockScale=off, RndMeth=Zero, SaturateOnIntegerOverflow=off}
      mask prompts: Inputs "Number of input ports:"; ZeroCross "Enable zero-crossing detection"; SampleTime "Sample time (-1 for inherited):"; InputSameDT "Require all inputs to have the same data type"; OutMin "Output minimum:"; OutMax "Output maximum:"; OutDataTypeStr "Output data type:"; LockScale "Lock output data type setting against changes by the fixed-point tools"; RndMeth "Integer rounding mode:"; SaturateOnIntegerOverflow "Saturate on integer overflow"
      mask help: Output min or max of input. For a single input, operators are applied across the input vector. For multiple inputs, operators are applied across the inputs.
      mask Help: web([fileparts(which('Lib_built')) filesep 'hlp' filesep 'lib_MinMax' '.html'], '-helpbrowser')
      mask TypeOptions Function: Function
      mask TypeOptions Inputs: Inputs
      mask TypeOptions ZeroCross: ZeroCross
      mask TypeOptions SampleTime: SampleTime
      mask TypeOptions InputSameDT: InputSameDT
      mask TypeOptions OutMin: OutMin
      mask TypeOptions OutMax: OutMax
      mask TypeOptions OutDataTypeStr: OutDataTypeStr
      mask TypeOptions LockScale: LockScale
      mask TypeOptions RndMeth: RndMeth
      mask TypeOptions SaturateOnIntegerOverflow: SaturateOnIntegerOverflow
  MinMax1 : MinMax  Tag=Controls_Lib_V1.0  Function=max  Inputs=Inputs  OutMin=OutMin  OutMax=OutMax  OutDataTypeStr=single  RndMeth=Zero  SampleTime=SampleTime  InputSameDT=on  mask(MinMax){Function=max, Inputs=2, ZeroCross=on, SampleTime=-1, InputSameDT=on, OutMin=[], OutMax=[], OutDataTypeStr=single, LockScale=off, RndMeth=Zero, SaturateOnIntegerOverflow=off}
      mask prompts: Inputs "Number of input ports:"; ZeroCross "Enable zero-crossing detection"; SampleTime "Sample time (-1 for inherited):"; InputSameDT "Require all inputs to have the same data type"; OutMin "Output minimum:"; OutMax "Output maximum:"; OutDataTypeStr "Output data type:"; LockScale "Lock output data type setting against changes by the fixed-point tools"; RndMeth "Integer rounding mode:"; SaturateOnIntegerOverflow "Saturate on integer overflow"
      mask help: Output min or max of input. For a single input, operators are applied across the input vector. For multiple inputs, operators are applied across the inputs.
      mask Help: web([fileparts(which('Lib_built')) filesep 'hlp' filesep 'lib_MinMax' '.html'], '-helpbrowser')
      mask TypeOptions Function: Function
      mask TypeOptions Inputs: Inputs
      mask TypeOptions ZeroCross: ZeroCross
      mask TypeOptions SampleTime: SampleTime
      mask TypeOptions InputSameDT: InputSameDT
      mask TypeOptions OutMin: OutMin
      mask TypeOptions OutMax: OutMax
      mask TypeOptions OutDataTypeStr: OutDataTypeStr
      mask TypeOptions LockScale: LockScale
      mask TypeOptions RndMeth: RndMeth
      mask TypeOptions SaturateOnIntegerOverflow: SaturateOnIntegerOverflow
  RelationalOperator : RelationalOperator  Tag=Controls_Lib_V1.0  Operator=~=  OutDataTypeStr=boolean  SampleTime=SampleTime  RndMeth=Nearest  InputSameDT=on  mask(Relational operator){Operator=~=, ZeroCross=on, SampleTime=-1, InputSameDT=on, OutDataTypeStr=boolean}
      mask prompts: Operator "Relational operator:"; ZeroCross "Enable zero-crossing detection"; SampleTime "Sample time (-1 for inherited):"; InputSameDT "Require all inputs to have the same data type"; OutDataTypeStr "Output data type:"
      mask help: Applies the selected relational operator to the inputs and outputs the result. The top (or left) input corresponds to the first operand.
      mask Help: web([fileparts(which('Lib_built')) filesep 'hlp' filesep 'lib_Relational' '.html'], '-helpbrowser')
      mask TypeOptions Operator: Operator
      mask TypeOptions ZeroCross: ZeroCross
      mask TypeOptions SampleTime: SampleTime
      mask TypeOptions InputSameDT: InputSameDT
      mask TypeOptions OutDataTypeStr: OutDataTypeStr
  ValSat : Outport  Tag=Controls_Lib_V1.0  OutDataTypeStr=single  InitialOutput=0
  IsSat : Outport  Tag=Controls_Lib_V1.0  Port=2  OutDataTypeStr=boolean  InitialOutput=0
  wires:
  Max/1 -> MinMax/1
  Inp/1 -> MinMax/2, RelationalOperator/2
  MinMax/1 -> MinMax1/1
  Min/1 -> MinMax1/2
  MinMax1/1 -> RelationalOperator/1, ValSat/1
  RelationalOperator/1 -> IsSat/1
